simulink model "controller"  (R2022b)
settings: Solver=FixedStepAuto  StartTime=0.0  StopTime=10.0  FixedStep=1/100  RelTol=1e-3
undefined symbols (not defined in the file or in its folder): MAX_TORQUE, MAX_TORQUE_REVERSE
libraries: slpidlib x1
settings Model: Creator=DAUIN-Win10  LastModifiedBy=David
settings DebuggingCC: UnconnectedInputMsg=warning  UnconnectedOutputMsg=warning  UnconnectedLineMsg=warning
settings ModelReferenceCC: EnableRefExpFcnMdlSchedulingChecks=on
settings RTWCC: DLArmComputeVersion=19.05

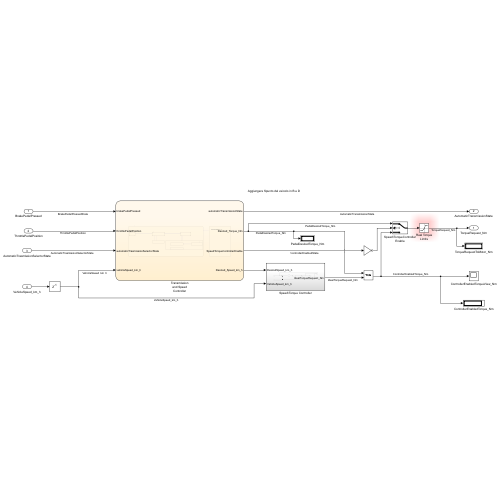
[thumbnail: Simulink's stored preview of the top-level diagram]
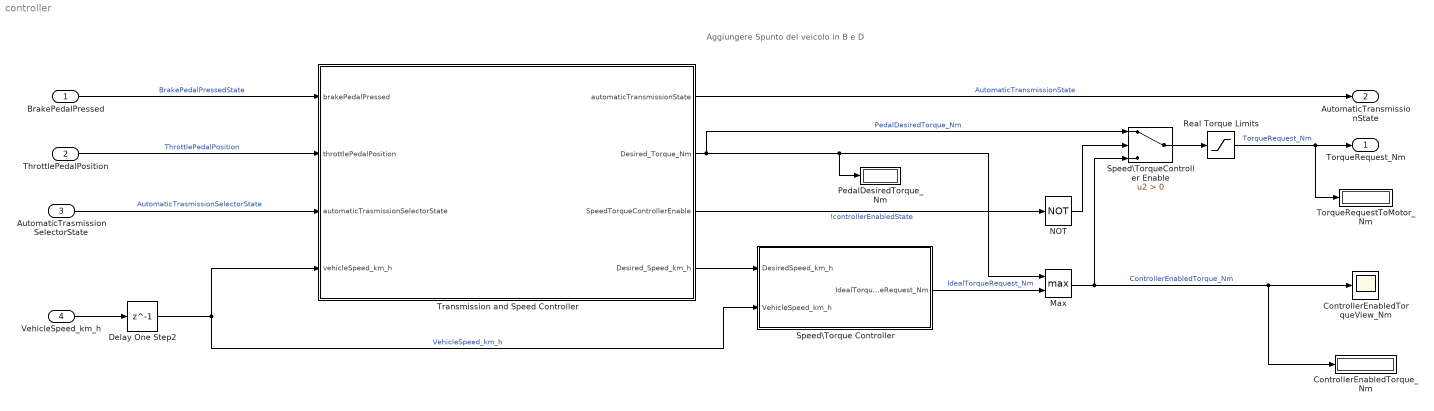
== system controller ==
  note: Aggiungere Spunto del veicolo in B e D
  BrakePedalPressed : Inport  OutDataTypeStr=boolean
  ThrottlePedalPosition : Inport  Port=2  OutDataTypeStr=single
  AutomaticTrasmissionSelectorState : Inport  Port=3  OutDataTypeStr=Enum: TransmissionState
  VehicleSpeed_km_h : Inport  Port=4  OutDataTypeStr=single  Unit=km/h
  ControllerEnabledTorqueView_Nm : Scope
  ControllerEnabledTorque_Nm : Display
  Delay One Step2 : Delay  DelayLength=1  SampleTime=1/100
  Max : MinMax  Function=max  Inputs=2
  NOT : Logic  Operator=NOT  IconShape=distinctive  AllPortsSameDT=off  OutDataTypeStr=boolean
  PedalDesiredTorque_Nm : Display
  Real Torque Limits : Saturate  UpperLimit=MAX_TORQUE  LowerLimit=-MAX_TORQUE_REVERSE
  Speed\Torque Controller : Subsystem
  Speed\TorqueController Enable : Switch  Criteria=u2 > Threshold  SaturateOnIntegerOverflow=off  InputSameDT=off
  TorqueRequestToMotor_Nm : Display
  Transmission and Speed Controller : Stateflow chart  TreatAsAtomicUnit=on
  TorqueRequest_Nm : Outport  OutDataTypeStr=single  Unit=N*m
  AutomaticTransmissionState : Outport  Port=2  OutDataTypeStr=Enum: TransmissionState
  wires:
  Real Torque Limits/1 -> TorqueRequestToMotor_Nm/1, TorqueRequest_Nm/1  "TorqueRequest_Nm"
  AutomaticTrasmissionSelectorState/1 -> Transmission and Speed Controller/3(automaticTrasmissionSelectorState)  "AutomaticTrasmissionSelectorState"
  ThrottlePedalPosition/1 -> Transmission and Speed Controller/2(throttlePedalPosition)  "ThrottlePedalPosition"
  Speed\Torque Controller/1(IdealTorqueRequest_Nm) -> Max/2  "IdealTorqueRequest_Nm"
  Transmission and Speed Controller/4(Desired_Speed_km_h) -> Speed\Torque Controller/1(DesiredSpeed_km_h)
  Transmission and Speed Controller/3(SpeedTorqueControllerEnable) -> NOT/1  "!controllerEnabledState"
  BrakePedalPressed/1 -> Transmission and Speed Controller/1(brakePedalPressed)  "BrakePedalPressedState"
  Delay One Step2/1 -> Speed\Torque Controller/2(VehicleSpeed_km_h), Transmission and Speed Controller/4(vehicleSpeed_km_h)  "VehicleSpeed_km_h"
  Transmission and Speed Controller/1(automaticTransmissionState) -> AutomaticTransmissionState/1  "AutomaticTransmissionState"
  Speed\TorqueController Enable/1 -> Real Torque Limits/1
  Transmission and Speed Controller/2(Desired_Torque_Nm) -> Max/1, PedalDesiredTorque_Nm/1, Speed\TorqueController Enable/1  "PedalDesiredTorque_Nm"
  VehicleSpeed_km_h/1 -> Delay One Step2/1
  Max/1 -> ControllerEnabledTorque_Nm/1, ControllerEnabledTorqueView_Nm/1, Speed\TorqueController Enable/3  "ControllerEnabledTorque_Nm"
  NOT/1 -> Speed\TorqueController Enable/2

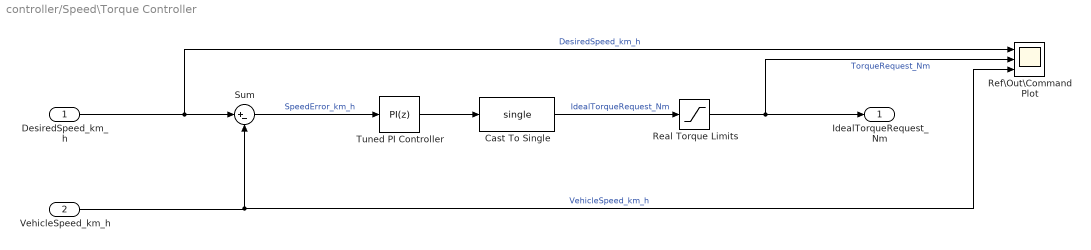
== system controller/Speed\Torque Controller ==
  DesiredSpeed_km_h : Inport
  VehicleSpeed_km_h : Inport  Port=2
  Cast To Single : DataTypeConversion  OutDataTypeStr=single  SaturateOnIntegerOverflow=off  RndMeth=Floor
  Real Torque Limits : Saturate  UpperLimit=MAX_TORQUE  LowerLimit=-MAX_TORQUE_REVERSE
  Ref\Out\Command Plot : Scope  NumInputPorts=3
  Sum : Sum  Inputs=|+-
  Tuned PI Controller : slpidlib/PID Controller  Controller=PI  Form=Parallel  TimeDomain=Discrete-time  UseExternalTs=off  SampleTime=1/100  IntegratorMethod=Forward Euler  FilterMethod=Forward Euler  ControllerParametersSource=internal  P=79.689863897109  I=82.1622460012644  UseKiTs=off  D=2.01264569507152  N=1.91388047645984  UseFilter=on  TunerSelectOption=Transfer Function Based (PID Tuner App)  InitialConditionSource=internal  InitialConditionForIntegrator=0  InitialConditionForFilter=0  DifferentiatorICPrevScaledInput=0  ExternalReset=none  TrackingMode=off  Kt=1  LimitOutput=off  SatLimitsSource=internal  UpperSaturationLimit=MAX_TORQUE  LowerSaturationLimit=-MAX_TORQUE_REVERSE  LinearizeAsGain=on  AntiWindupMode=none  Kb=1  LimitIntegrator=on  UpperIntegratorSaturationLimit=MAX_TORQUE  LowerIntegratorSaturationLimit=-MAX_TORQUE_REVERSE  POutMin=[]  POutMax=[]  IOutMin=[]  IOutMax=[]  DOutMin=[]  DOutMax=[]  NOutMin=[]  NOutMax=[]  SumOutMin=[]  SumOutMax=[]  SaturationOutMin=[]  SaturationOutMax=[]  PParamMin=[]  PParamMax=[]  IParamMin=[]  IParamMax=[]  DParamMin=[]  DParamMax=[]  NParamMin=[]  NParamMax=[]  KbParamMin=[]  KbParamMax=[]  KtParamMin=[]  KtParamMax=[]  KbOutMin=[]  KbOutMax=[]  KtOutMin=[]  KtOutMax=[]  IntegratorOutMin=[]  IntegratorOutMax=[]  FilterOutMin=[]  FilterOutMax=[]  SumI1OutMin=[]  SumI1OutMax=[]  SumI2OutMin=[]  SumI2OutMax=[]  SumI3OutMin=[]  SumI3OutMax=[]  SumI4OutMin=[]  SumI4OutMax=[]  SumDOutMin=[]  SumDOutMax=[]  DifferentiatorOutMin=[]  DifferentiatorOutMax=[]  FilterDiffOutCoefMin=[]  FilterDiffOutCoefMax=[]  ReciprocalOutMin=[]  ReciprocalOutMax=[]  SumDenOutMin=[]  SumDenOutMax=[]  SumNumOutMin=[]  SumNumOutMax=[]  DivideOutMin=[]  DivideOutMax=[]  UdiffTsProdOutMin=[]  UdiffTsProdOutMax=[]  NTsProdOutMin=[]  NTsProdOutMax=[]  UintegralTsProdOutMin=[]  UintegralTsProdOutMax=[]  UngainTsProdOutMin=[]  UngainTsProdOutMax=[]  ClampingZeroOutDataTypeStr=Inherit: Inherit via back propagation  ClampingZeroOutMin=[]  ClampingZeroOutMax=[]  FilterDenConstantOutDataTypeStr=Inherit: Inherit via back propagation  FilterDenConstantOutMin=[]  FilterDenConstantOutMax=[]  PCopyOutDataTypeStr=Inherit: Inherit via back propagation  PCopyOutMin=[]  PCopyOutMax=[]  NCopyOutDataTypeStr=Inherit: Inherit via back propagation  NCopyOutMin=[]  NCopyOutMax=[]  IntegratorContinuousStateAttributes=''  IntegratorStateMustResolveToSignalObject=off  IntegratorRTWStateStorageClass=Auto  FilterContinuousStateAttributes=''  FilterStateMustResolveToSignalObject=off  FilterRTWStateStorageClass=Auto  ParallelPVariant=InternalParameters  IdealPVariant=Disabled  IVariant=InternalParameters  DVariant=Disabled  IntegratorVariant=Discrete  SatVariant=Disabled  AWVariant=Passthrough  PCopyVariant=Disabled  TRVariant=Disabled  FdbkBlocksVariant=Forward  IdealPFdbkVariant=Disabled  SatFdbkVariant=Disabled  DerivativeFilterVariant=Disabled  NVariant=Disabled  NCopyVariant=Disabled_SignalSpec  FilterICVariant=Disabled  IntegratorICVariant=InternalICs  ExternalResetVariant=Disabled  TRSumVariant=Passthrough  SumFdbkVariant=Disabled  SumVariant=Sum_PI  TsampFilterVariant=InternalTs  TsampNgainVariant=Passthrough  TsampIntegralVariant=Passthrough  ExternalSaturationOutDataTypeStr=Inherit: Same as second input
  IdealTorqueRequest_Nm : Outport
  wires:
  Cast To Single/1 -> Real Torque Limits/1  "IdealTorqueRequest_Nm"
  Tuned PI Controller/1 -> Cast To Single/1
  DesiredSpeed_km_h/1 -> Ref\Out\Command Plot/1, Sum/1  "DesiredSpeed_km_h"
  VehicleSpeed_km_h/1 -> Ref\Out\Command Plot/3, Sum/2  "VehicleSpeed_km_h"
  Sum/1 -> Tuned PI Controller/1  "SpeedError_km_h"
  Real Torque Limits/1 -> Ref\Out\Command Plot/2, IdealTorqueRequest_Nm/1  "TorqueRequest_Nm"

== stateflow chart controller/Transmission and Speed Controller ==
  state Working
    state Park
      entry:
      automaticTransmissionState=Park;
      during:
      SpeedTorqueControllerEnable=0;
      Desired_Torque_Nm=0;
      %activate EHandbrake
    state Neutral
      entry:
      automaticTransmissionState=Neutral;
      during:
      Desired_Torque_Nm=0;
      SpeedTorqueControllerEnable=0;
    state Drive
      entry:
      automaticTransmissionState=Drive;
      during:
      Desired_Torque_Nm=throttlePedalPosition*MAX_TORQUE;
      SpeedTorqueControllerEnable=0;
    state Reverse
      entry:
      automaticTransmissionState=Reverse;
      during:
      Desired_Torque_Nm=-throttlePedalPosition*MAX_REVERSE_TORQUE;
      SpeedTorqueControllerEnable=0;
    state Brake
      entry:
      automaticTransmissionState=Brake;
      state RegenerativeBraking
        during:
        Desired_Torque_Nm=-MAX_REVERSE_TORQUE*(1-3*throttlePedalPosition);
        Desired_Speed_km_h=0;
        SpeedTorqueControllerEnable=1;
      state Acceleration
        during:
        Desired_Torque_Nm=MAX_TORQUE*3/2*(throttlePedalPosition-1/3);
        SpeedTorqueControllerEnable=0;
      state LowSpeed
        during:
        Desired_Torque_Nm=-MAX_TORQUE*(1-3*throttlePedalPosition);
        Desired_Speed_km_h=0;
        SpeedTorqueControllerEnable=1;
      (default) -> Acceleration
      Acceleration -> RegenerativeBraking : [throttlePedalPosition<1/3]
      RegenerativeBraking -> Acceleration : [throttlePedalPosition>=1/3]
    (default) -> Neutral
    Neutral -> Drive [order 1] : [automaticTrasmissionSelectorState>=3&&brakePedalPressed==true&&vehicleSpeed_km_h>-5]
    Neutral -> Park [order 2] : [automaticTrasmissionSelectorState==0&&brakePedalPressed==true&&abs(vehicleSpeed_km_h)<=5]
    Drive -> Neutral [order 2] : [automaticTrasmissionSelectorState<3]
    Park -> Neutral : [automaticTrasmissionSelectorState~=0&&brakePedalPressed==true]
    Neutral -> Reverse [order 3] : [automaticTrasmissionSelectorState==1&&brakePedalPressed==true&&vehicleSpeed_km_h<=5]
    Reverse -> Neutral : [automaticTrasmissionSelectorState~=1]
    Drive -> Brake [order 1] : [automaticTrasmissionSelectorState==4&&throttlePedalPosition>1/3]
    Brake -> Drive : [automaticTrasmissionSelectorState~=4]
  state Fault
    note: FAULTY CONTROL TO BE IMPLEMENTED LATER,
        | so this for now is an unreachable state
  (default) -> Working
  Working -> Fault : [fault==1]
  data: brakePedalPressed input; automaticTransmissionState output Enum: TransmissionState; fault local =0; throttlePedalPosition input single; automaticTrasmissionSelectorState input; vehicleSpeed_km_h input; MAX_TORQUE constant single =80; Desired_Torque_Nm output single; SpeedTorqueControllerEnable output; MAX_REVERSE_TORQUE constant single =40; Desired_Speed_km_h output
